simulink model "Drone_Simulation"  (R2020a)
settings: Solver=ode1  StartTime=0.0  StopTime=50  FixedStep=1e-3
values from neighbouring files (symbols this model uses):
  AeEMSC = 1    [Qball_X8_Model.m]
  alpha1TDDBSC = 1    [Qball_X8_Model.m]    (also in ReliabilityModel_Script.m = 0.7)
  bBNG = 1.2    [ReliabilityModel_Script.m]
  bEMSC = 1    [Qball_X8_Model.m]
  bEVCAP = 1    [Qball_X8_Model.m]    (also in ReliabilityModel_Script.m = 1.1)
  BNG_Motor1 = 0.8    [ReliabilityModel_Script.m]
  BNG_Motor2 = 1    [ReliabilityModel_Script.m]
  BNG_Motor3 = 1    [ReliabilityModel_Script.m]
  BNG_Motor4 = 1    [ReliabilityModel_Script.m]
  BNG_Motor5 = 1    [ReliabilityModel_Script.m]
  BNG_Motor6 = 1    [ReliabilityModel_Script.m]
  bp = 0.001    [ControlLawsScript.m]    (also in ControlLaws_Script.m)
  bq = 0.001    [ControlLawsScript.m]    (also in ControlLaws_Script.m)
  br = 0.001    [ControlLawsScript.m]    (also in ControlLaws_Script.m)
  bTDDBSC = 1    [Qball_X8_Model.m]    (also in ReliabilityModel_Script.m = 1.1)
  bWDG = 1    [Qball_X8_Model.m]    (also in ReliabilityModel_Script.m = 1.1)
  C_A = [     k_T           k_T          k_T                k_T          k_T         k_T ... (first row only)    [ControlLawsScript.m]    (also in ControlLaws_Script.m)
  C_mot = 1    [Qball_X8_Model.m]    (also in ReliabilityModel_Script.m = 17.46)
  C_th_esc = 1    [Qball_X8_Model.m]    (also in ReliabilityModel_Script.m = 1.67)
  CAPEV_Motor1 = 0.8    [ReliabilityModel_Script.m]
  CAPEV_Motor2 = 1    [ReliabilityModel_Script.m]
  CAPEV_Motor3 = 1    [ReliabilityModel_Script.m]
  CAPEV_Motor4 = 1    [ReliabilityModel_Script.m]
  CAPEV_Motor5 = 1    [ReliabilityModel_Script.m]
  CAPEV_Motor6 = 1    [ReliabilityModel_Script.m]
  cdx = cx*m    (= 17.4057414746)    [ControlLawsScript.m]    (also in ControlLaws_Script.m)
  cdy = cy*m    (= 17.4057414746)    [ControlLawsScript.m]    (also in ControlLaws_Script.m)
  cdz = cz*m    (= 17.4057414746)    [ControlLawsScript.m]    (also in ControlLaws_Script.m)
  EaEMSC = 1    [Qball_X8_Model.m]
  EaEVCAP = 1    [Qball_X8_Model.m]    (also in ReliabilityModel_Script.m = 0.94)
  EalphaTDDBSC = 1    [Qball_X8_Model.m]    (also in ReliabilityModel_Script.m = 0.7)
  EaTDDBSC = 1    [Qball_X8_Model.m]    (also in ReliabilityModel_Script.m = 0.7)
  EaWDG = 1    [Qball_X8_Model.m]    (also in ReliabilityModel_Script.m = 0.5)
  g = 9.80665    [ControlLawsScript.m]    (also in ControlLaws_Script.m; Qball_X8_Model.m = 9.87)
  JrefEMSC = 1    [Qball_X8_Model.m]
  Jz = 0.15887270137511    (= 0.158872701375)    [ControlLawsScript.m]    (also in ControlLaws_Script.m)
  k_b = 1    [Qball_X8_Model.m]    (also in ReliabilityModel_Script.m = -21.8546)
  Kp = (Jx/Tc)-bp    (= 4.11390529802)    [ControlLawsScript.m]    (also in ControlLaws_Script.m)
  Kp2 = Jx*((4/ts))*((-4/ts)+((bp+Kp)/Jx))/Kp    (= 6.72163348437)    [ControlLawsScript.m]    (also in ControlLaws_Script.m)
  Kq = (Jy/Tc)-bq    (= 4.12186008142)    [ControlLawsScript.m]    (also in ControlLaws_Script.m)
  Kq2 = Jy*((4/ts))*((-4/ts)+((bq+Kq)/Jy))/Kq    (= 6.72163033191)    [ControlLawsScript.m]    (also in ControlLaws_Script.m)
  Kr = (Jz/(tsy/25))-br    (= 7.94263506876)    [ControlLawsScript.m]    (also in ControlLaws_Script.m)
  Kr2 = Jz*((4/tsy))*((-4/tsy)+((br+Kr)/Jz))/Kr    (= 6.72084606682)    [ControlLawsScript.m]    (also in ControlLaws_Script.m)
  kv = 1/930    (= 0.0010752688172)    [StingerScript.m]
  Kx = abs(Kx)    [ControlLawsScript.m]    (also in ControlLaws_Script.m)
  Ky = abs(Ky)    [ControlLawsScript.m]    (also in ControlLaws_Script.m)
  Kz = (m/Tcz)-cz    (= 38.5143536865)    [ControlLawsScript.m]    (also in ControlLaws_Script.m)
  Kz2 = m*((4/tsz))*((-4/tsz)+((cz+Kz)/m))/Kz    (= 1.89810050529)    [ControlLawsScript.m]    (also in ControlLaws_Script.m)
  LnomEMSC = 1    [Qball_X8_Model.m]
  LnomEVCAP = 1    [Qball_X8_Model.m]    (also in ReliabilityModel_Script.m = 10800000)
  LnomTDDBSC = 1    [Qball_X8_Model.m]    (also in ReliabilityModel_Script.m = 9997200)
  LnomWDG = 1    [Qball_X8_Model.m]    (also in ReliabilityModel_Script.m = 72000000)
  m = 3.4811482949175    (= 3.48114829492)    [ControlLawsScript.m]    (also in ControlLaws_Script.m; Qball_X8_Model.m = 1.45)
  max_yaw_moment = k_y*hov_thrust/k_T    (= 0.323744079512)    [ControlLawsScript.m]    (also in ControlLaws_Script.m = 0.57666914163)
  NEMSC = 1    [Qball_X8_Model.m]
  nEVCAP = 1    [Qball_X8_Model.m]    (also in ReliabilityModel_Script.m)
  pconst = 2    [Qball_X8_Model.m]    (also in ReliabilityModel_Script.m)
  pitch_angle_limit = 32/R2D    (= 0.558505360638)    [ControlLawsScript.m]    (also in ControlLaws_Script.m)
  R2D = 180/pi    (= 57.2957795131)    [ControlLawsScript.m]    (also in ControlLaws_Script.m)
  R_th_esc = 1    [Qball_X8_Model.m]    (also in ReliabilityModel_Script.m = 5.14)
  R_th_mot = 1    [Qball_X8_Model.m]    (also in ReliabilityModel_Script.m = 8.59)
  Re = 0.008    [Qball_X8_Model.m]    (also in ReliabilityModel_Script.m)
  roll_angle_limit = 32/R2D    (= 0.558505360638)    [ControlLawsScript.m]    (also in ControlLaws_Script.m)
  RrefBNG = 0.9    [ReliabilityModel_Script.m]
  RrefEMSC = 1    [Qball_X8_Model.m]
  RrefEVCAP = 1    [Qball_X8_Model.m]    (also in ReliabilityModel_Script.m = 0.9)
  RrefTDDBSC = 1    [Qball_X8_Model.m]    (also in ReliabilityModel_Script.m = 0.37)
  RrefWDG = 1    [Qball_X8_Model.m]    (also in ReliabilityModel_Script.m = 0.98)
  SCTDDB_Motor1 = 0.8    [ReliabilityModel_Script.m]
  SCTDDB_Motor2 = 1    [ReliabilityModel_Script.m]
  SCTDDB_Motor3 = 1    [ReliabilityModel_Script.m]
  SCTDDB_Motor4 = 1    [ReliabilityModel_Script.m]
  SCTDDB_Motor5 = 1    [ReliabilityModel_Script.m]
  SCTDDB_Motor6 = 1    [ReliabilityModel_Script.m]
  T_amb = 1    [Qball_X8_Model.m]    (also in ReliabilityModel_Script.m = 20)
  T_amb_mot = 1    [Qball_X8_Model.m]    (also in ReliabilityModel_Script.m = 20)
  t_D_SCTDDB = 30    [ReliabilityModel_Script.m]
  TrefEMSC = 1    [Qball_X8_Model.m]
  TrefEVCAP = 1    [Qball_X8_Model.m]    (also in ReliabilityModel_Script.m = 105)
  TrefTDDBSC = 1    [Qball_X8_Model.m]    (also in ReliabilityModel_Script.m = 150)
  TrefWDG = 1    [Qball_X8_Model.m]    (also in ReliabilityModel_Script.m = 40)
  Ub = 12    [Qball_X8_Model.m]    (also in ReliabilityModel_Script.m)
  VmaxEVCAP = 1    [Qball_X8_Model.m]    (also in ReliabilityModel_Script.m = 35)
  VnomEVCAP = 1    [Qball_X8_Model.m]    (also in ReliabilityModel_Script.m = 35)
  WDG_Motor1 = 0.8    [ReliabilityModel_Script.m]
  WDG_Motor2 = 1    [ReliabilityModel_Script.m]
  WDG_Motor3 = 1    [ReliabilityModel_Script.m]
  WDG_Motor4 = 1    [ReliabilityModel_Script.m]
  WDG_Motor5 = 1    [ReliabilityModel_Script.m]
  WDG_Motor6 = 1    [ReliabilityModel_Script.m]
  z_x = cx    (= 5)    [ControlLawsScript.m]    (also in ControlLaws_Script.m)
  z_y = cy    (= 5)    [ControlLawsScript.m]    (also in ControlLaws_Script.m)
undefined symbols (not defined in the file or in its folder): FuselageContactForces, LeftAftArm, LeftAftSkid, LeftArm, LeftFrontArm, LeftFrontSkid, LeftSideContactForces, Lower, missionPlanX, missionPlanY, missionPlanYaw, missionPlanZ, Newton, Raphson, RightAftArm, RightAftSkid, RightArm, RightFrontArm, RightFrontSkid, RightSideContactForces, SkidsContactForces, timeConstant, Upper, X, Y, Z
libraries: sm_lib x90, nesl_utility x78, fl_lib x61, ee_lib x19, dspinverses x1, dspmtrx3 x1
(part 5 of 5)

== system Drone_Simulation/PLANT MODEL/PROPELLER AND ARMS/Arms ==
  Arm {1..6} (6 alike) : sm_lib/Body Elements/File Solid  ExtGeomFileName=STL files\Arm.stl  UnitType=Custom  ExtGeomFileUnits=mm  StepReaderType=HEX  ExportConvexHullGeometry=on  InertiaType=CalculateFromGeometry  Mass=1  MassUnits=kg  CenterOfMass=[0 0 0]  CenterOfMassUnits=m  MomentsOfInertia=[1 1 1]  MomentsOfInertiaUnits=kg*m^2  ProductsOfInertia=[0 0 0]  ProductsOfInertiaUnits=kg*m^2  BasedOnType=Density  Density=rho1  DensityUnits=kg/m^3  DoExposeReferenceFrame=on  SerializedFrames=<Frames/>  GraphicType=FromGeometry  MarkerShape=Sphere  MarkerSize=10  GraphicVisPropType=SimpleVisualProperties  GraphicDiffuseColor=rgb1  GraphicSpecularColor=[0.5 0.5 0.5 1.0]  GraphicAmbientColor=[0.15 0.15 0.15 1.0]  GraphicEmissiveColor=[0.0 0.0 0.0 1.0]  GraphicShininess=75  GraphicOpacity=op1
  Left Contact Arms : SimscapeBus  HierarchyStrings=LeftFrontArm;LeftArm;LeftAftArm
  Motor {1..6} (6 alike) : sm_lib/Body Elements/File Solid  ExtGeomFileName=STL files\Motor.stp  UnitType=FromFile  ExtGeomFileUnits=mm  StepReaderType=HEX  ExportConvexHullGeometry=off  InertiaType=CalculateFromGeometry  Mass=1  MassUnits=kg  CenterOfMass=[0 0 0]  CenterOfMassUnits=m  MomentsOfInertia=[1 1 1]  MomentsOfInertiaUnits=kg*m^2  ProductsOfInertia=[0 0 0]  ProductsOfInertiaUnits=kg*m^2  BasedOnType=Density  Density=rhoM  DensityUnits=kg/m^3  DoExposeReferenceFrame=on  SerializedFrames=<Frames/>  GraphicType=FromGeometry  MarkerShape=Sphere  MarkerSize=10  GraphicVisPropType=SimpleVisualProperties  GraphicDiffuseColor=[0.5 0.5 0.5]  GraphicSpecularColor=[0.5 0.5 0.5 1.0]  GraphicAmbientColor=[0.15 0.15 0.15 1.0]  GraphicEmissiveColor=[0.0 0.0 0.0 1.0]  GraphicShininess=75  GraphicOpacity=1.0
  Right Contact Arms : SimscapeBus  HierarchyStrings=RightFrontArm;RightArm;RightAftArm
  Rigid Transform{,6..10} (6 alike) : sm_lib/Frames and Transforms/Rigid Transform  TranslationMethod=Cartesian  TranslationStandardOffset=0  TranslationLengthUnit=m  TranslationStandardAxis=+Z  TranslationCartesianOffset=[0 0.3805 0.017]  TranslationROffset=0  TranslationROffsetUnits=m  TranslationZOffset=0  TranslationZOffsetUnits=m  TranslationThetaOffset=0  TranslationThetaOffsetUnits=deg  RotationMethod=StandardAxis  RotationAngleUnits=deg  RotationStandardAxis=-X  RotationAngle=180  RotationArbitraryAxis=[0 0 1]  FollAlignAxisA=+X  BaseAlignAxisA=+Y  FollAlignAxisB=+Y  BaseAlignAxisB=+Z  RotationSequenceAxes=FollowerAxes  RotationSequence=XYX  RotationSequenceAngles=[0 0 0]  RotationSequenceAnglesUnits=deg  RotationMatrix=[1 0 0; 0 1 0; 0 0 1]
  Rigid Transform1 : sm_lib/Frames and Transforms/Rigid Transform  TranslationMethod=Cartesian  TranslationStandardOffset=0  TranslationLengthUnit=m  TranslationStandardAxis=+Z  TranslationCartesianOffset=[0 0 0]  TranslationROffset=0  TranslationROffsetUnits=m  TranslationZOffset=0  TranslationZOffsetUnits=m  TranslationThetaOffset=0  TranslationThetaOffsetUnits=deg  RotationMethod=StandardAxis  RotationAngleUnits=deg  RotationStandardAxis=+Z  RotationAngle=0  RotationArbitraryAxis=[0 0 1]  FollAlignAxisA=+X  BaseAlignAxisA=+Y  FollAlignAxisB=+Y  BaseAlignAxisB=+Z  RotationSequenceAxes=FollowerAxes  RotationSequence=ZYX  RotationSequenceAngles=[0 0 0]  RotationSequenceAnglesUnits=deg  RotationMatrix=[1 0 0; 0 1 0; 0 0 1]
  Rigid Transform2 : sm_lib/Frames and Transforms/Rigid Transform  TranslationMethod=Cartesian  TranslationStandardOffset=0  TranslationLengthUnit=m  TranslationStandardAxis=+Z  TranslationCartesianOffset=[0 0 0]  TranslationROffset=0  TranslationROffsetUnits=m  TranslationZOffset=0  TranslationZOffsetUnits=m  TranslationThetaOffset=0  TranslationThetaOffsetUnits=deg  RotationMethod=StandardAxis  RotationAngleUnits=deg  RotationStandardAxis=+Z  RotationAngle=60  RotationArbitraryAxis=[0 0 1]  FollAlignAxisA=+X  BaseAlignAxisA=+Y  FollAlignAxisB=+Y  BaseAlignAxisB=+Z  RotationSequenceAxes=FollowerAxes  RotationSequence=ZYX  RotationSequenceAngles=[0 0 0]  RotationSequenceAnglesUnits=deg  RotationMatrix=[1 0 0; 0 1 0; 0 0 1]
  Rigid Transform3 : sm_lib/Frames and Transforms/Rigid Transform  TranslationMethod=Cartesian  TranslationStandardOffset=0  TranslationLengthUnit=m  TranslationStandardAxis=+Z  TranslationCartesianOffset=[0 0 0]  TranslationROffset=0  TranslationROffsetUnits=m  TranslationZOffset=0  TranslationZOffsetUnits=m  TranslationThetaOffset=0  TranslationThetaOffsetUnits=deg  RotationMethod=StandardAxis  RotationAngleUnits=deg  RotationStandardAxis=+Z  RotationAngle=120  RotationArbitraryAxis=[0 0 1]  FollAlignAxisA=+X  BaseAlignAxisA=+Y  FollAlignAxisB=+Y  BaseAlignAxisB=+Z  RotationSequenceAxes=FollowerAxes  RotationSequence=ZYX  RotationSequenceAngles=[0 0 0]  RotationSequenceAnglesUnits=deg  RotationMatrix=[1 0 0; 0 1 0; 0 0 1]
  Rigid Transform4 : sm_lib/Frames and Transforms/Rigid Transform  TranslationMethod=Cartesian  TranslationStandardOffset=0  TranslationLengthUnit=m  TranslationStandardAxis=+Z  TranslationCartesianOffset=[0 0 0]  TranslationROffset=0  TranslationROffsetUnits=m  TranslationZOffset=0  TranslationZOffsetUnits=m  TranslationThetaOffset=0  TranslationThetaOffsetUnits=deg  RotationMethod=StandardAxis  RotationAngleUnits=deg  RotationStandardAxis=+Z  RotationAngle=180  RotationArbitraryAxis=[0 0 1]  FollAlignAxisA=+X  BaseAlignAxisA=+Y  FollAlignAxisB=+Y  BaseAlignAxisB=+Z  RotationSequenceAxes=FollowerAxes  RotationSequence=ZYX  RotationSequenceAngles=[0 0 0]  RotationSequenceAnglesUnits=deg  RotationMatrix=[1 0 0; 0 1 0; 0 0 1]
  Rigid Transform5 : sm_lib/Frames and Transforms/Rigid Transform  TranslationMethod=Cartesian  TranslationStandardOffset=0  TranslationLengthUnit=m  TranslationStandardAxis=+Z  TranslationCartesianOffset=[0 0 0]  TranslationROffset=0  TranslationROffsetUnits=m  TranslationZOffset=0  TranslationZOffsetUnits=m  TranslationThetaOffset=0  TranslationThetaOffsetUnits=deg  RotationMethod=StandardAxis  RotationAngleUnits=deg  RotationStandardAxis=+Z  RotationAngle=240  RotationArbitraryAxis=[0 0 1]  FollAlignAxisA=+X  BaseAlignAxisA=+Y  FollAlignAxisB=+Y  BaseAlignAxisB=+Z  RotationSequenceAxes=FollowerAxes  RotationSequence=ZYX  RotationSequenceAngles=[0 0 0]  RotationSequenceAnglesUnits=deg  RotationMatrix=[1 0 0; 0 1 0; 0 0 1]
  Rigid Transform62 : sm_lib/Frames and Transforms/Rigid Transform  TranslationMethod=Cartesian  TranslationStandardOffset=0  TranslationLengthUnit=m  TranslationStandardAxis=+Z  TranslationCartesianOffset=[0 0 0]  TranslationROffset=0  TranslationROffsetUnits=m  TranslationZOffset=0  TranslationZOffsetUnits=m  TranslationThetaOffset=0  TranslationThetaOffsetUnits=deg  RotationMethod=StandardAxis  RotationAngleUnits=deg  RotationStandardAxis=+Z  RotationAngle=300  RotationArbitraryAxis=[0 0 1]  FollAlignAxisA=+X  BaseAlignAxisA=+Y  FollAlignAxisB=+Y  BaseAlignAxisB=+Z  RotationSequenceAxes=FollowerAxes  RotationSequence=ZYX  RotationSequenceAngles=[0 0 0]  RotationSequenceAnglesUnits=deg  RotationMatrix=[1 0 0; 0 1 0; 0 0 1]
  Left-Front : PMIOPort  Side=Left
  Right-Front : PMIOPort  Port=2  Side=Left
  Left : PMIOPort  Port=3  Side=Left
  Right : PMIOPort  Port=4  Side=Left
  Left-Aft : PMIOPort  Port=5  Side=Left
  Right-Aft : PMIOPort  Port=6  Side=Left
  Fuselage : PMIOPort  Port=7  Side=Left
  Left Contact : PMIOPort  Port=8  Side=Right
  Right Contact : PMIOPort  Port=9  Side=Right
  connections:
  Right-Front/RConn1 -- Arm 1/RConn1 -- Rigid Transform7/LConn1 -- Rigid Transform5/RConn1
  Left-Front/RConn1 -- Arm 6/RConn1 -- Rigid Transform10/LConn1 -- Rigid Transform62/RConn1
  Right-Aft/RConn1 -- Arm 3/RConn1 -- Rigid Transform/LConn1 -- Rigid Transform3/RConn1
  Left-Aft/RConn1 -- Arm 4/RConn1 -- Rigid Transform8/LConn1 -- Rigid Transform2/RConn1
  Left/RConn1 -- Rigid Transform1/RConn1 -- Arm 5/RConn1 -- Rigid Transform9/LConn1
  Rigid Transform1/LConn1 -- Rigid Transform62/LConn1 -- Rigid Transform5/LConn1 -- Rigid Transform4/LConn1 -- Rigid Transform3/LConn1 -- Rigid Transform2/LConn1 -- Fuselage/RConn1
  Right/RConn1 -- Arm 2/RConn1 -- Rigid Transform6/LConn1 -- Rigid Transform4/RConn1
  Right Contact/RConn1 -- Right Contact Arms/RConn1
  Arm 5/LConn1 -- Left Contact Arms/LConn2
  Arm 2/LConn1 -- Right Contact Arms/LConn2
  Arm 3/LConn1 -- Right Contact Arms/LConn3
  Arm 1/LConn1 -- Right Contact Arms/LConn1
  Arm 6/LConn1 -- Left Contact Arms/LConn1
  Arm 4/LConn1 -- Left Contact Arms/LConn3
  Left Contact/RConn1 -- Left Contact Arms/RConn1
  Motor 3/RConn1 -- Rigid Transform/RConn1
  Motor 2/RConn1 -- Rigid Transform6/RConn1
  Motor 1/RConn1 -- Rigid Transform7/RConn1
  Motor 4/RConn1 -- Rigid Transform8/RConn1
  Motor 5/RConn1 -- Rigid Transform9/RConn1
  Motor 6/RConn1 -- Rigid Transform10/RConn1

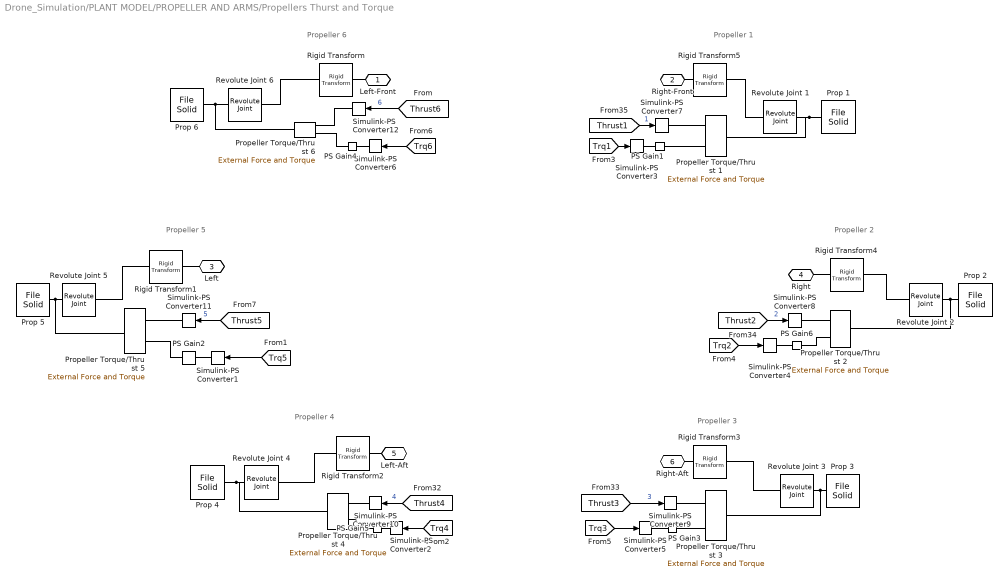
== system Drone_Simulation/PLANT MODEL/PROPELLER AND ARMS/Propellers Thurst and Torque ==
  note: Propeller 1
  note: Propeller 2
  note: Propeller 3
  note: Propeller 4
  note: Propeller 5
  note: Propeller 6
  PS Gain1 : fl_lib/Physical Signals/Functions/PS Gain  gain=-1
  PS Gain2 : fl_lib/Physical Signals/Functions/PS Gain  gain=-1
  PS Gain3 : fl_lib/Physical Signals/Functions/PS Gain  gain=-1
  PS Gain4 : fl_lib/Physical Signals/Functions/PS Gain  gain=1
  PS Gain5 : fl_lib/Physical Signals/Functions/PS Gain  gain=1
  PS Gain6 : fl_lib/Physical Signals/Functions/PS Gain  gain=1
  Prop {1..3,6} (4 alike) : sm_lib/Body Elements/File Solid  ExtGeomFileName=STL files\Propeller.stl  UnitType=Custom  ExtGeomFileUnits=m  StepReaderType=HEX  ExportConvexHullGeometry=off  InertiaType=CalculateFromGeometry  Mass=1  MassUnits=kg  CenterOfMass=[0 0 0]  CenterOfMassUnits=m  MomentsOfInertia=[1 1 1]  MomentsOfInertiaUnits=kg*m^2  ProductsOfInertia=[0 0 0]  ProductsOfInertiaUnits=kg*m^2  BasedOnType=Density  Density=rhoP  DensityUnits=kg/m^3  DoExposeReferenceFrame=on  SerializedFrames=<Frames/>  GraphicType=FromGeometry  MarkerShape=Sphere  MarkerSize=10  GraphicVisPropType=SimpleVisualProperties  GraphicDiffuseColor=rgbP  GraphicSpecularColor=[0.5 0.5 0.5 1.0]  GraphicAmbientColor=[0.15 0.15 0.15 1.0]  GraphicEmissiveColor=[0.0 0.0 0.0 1.0]  GraphicShininess=75  GraphicOpacity=opP
  Prop 4 : sm_lib/Body Elements/File Solid  ExtGeomFileName=STL files\Propeller.stl  UnitType=Custom  ExtGeomFileUnits=m  StepReaderType=HEX  ExportConvexHullGeometry=off  InertiaType=CalculateFromGeometry  Mass=1  MassUnits=kg  CenterOfMass=[0 0 0.1]  CenterOfMassUnits=m  MomentsOfInertia=[1 1 1]  MomentsOfInertiaUnits=kg*m^2  ProductsOfInertia=[0 0 0]  ProductsOfInertiaUnits=kg*m^2  BasedOnType=Density  Density=rhoP  DensityUnits=kg/m^3  DoExposeReferenceFrame=on  SerializedFrames=<Frames/>  GraphicType=FromGeometry  MarkerShape=Sphere  MarkerSize=10  GraphicVisPropType=SimpleVisualProperties  GraphicDiffuseColor=rgbP  GraphicSpecularColor=[0.5 0.5 0.5 1.0]  GraphicAmbientColor=[0.15 0.15 0.15 1.0]  GraphicEmissiveColor=[0.0 0.0 0.0 1.0]  GraphicShininess=75  GraphicOpacity=opP
  Prop 5 : sm_lib/Body Elements/File Solid  ExtGeomFileName=STL files\Propeller.stl  UnitType=Custom  ExtGeomFileUnits=m  StepReaderType=HEX  ExportConvexHullGeometry=off  InertiaType=CalculateFromGeometry  Mass=1  MassUnits=kg  CenterOfMass=[0 0 0.1]  CenterOfMassUnits=m  MomentsOfInertia=[1 1 1]  MomentsOfInertiaUnits=kg*m^2  ProductsOfInertia=[0 0 0]  ProductsOfInertiaUnits=kg*m^2  BasedOnType=Density  Density=rhoP  DensityUnits=kg/m^3  DoExposeReferenceFrame=on  SerializedFrames=<Frames/>  GraphicType=FromGeometry  MarkerShape=Sphere  MarkerSize=10  GraphicVisPropType=SimpleVisualProperties  GraphicDiffuseColor=rgbP  GraphicSpecularColor=[0.5 0.5 0.5 1.0]  GraphicAmbientColor=[0.15 0.15 0.15 1.0]  GraphicEmissiveColor=[0.0 0.0 0.0 1.0]  GraphicShininess=75  GraphicOpacity=opP
  Propeller Torque/Thrust {1..6} (6 alike) : sm_lib/Forces and Torques/External Force and Torque  ForceResolutionFrame=AttachedFrame  EnableForceX=off  EnableForceY=off  EnableForceZ=on  EnableForce=off  TorqueResolutionFrame=AttachedFrame  EnableTorqueX=off  EnableTorqueY=off  EnableTorqueZ=on  EnableTorque=off
  Revolute Joint {1..6} (6 alike) : sm_lib/Joints/Revolute Joint  JointMode=Normal  SenseConstraintForce=off  SenseConstraintForceX=off  SenseConstraintForceY=off  SenseConstraintForceZ=off  SenseConstraintTorque=off  SenseConstraintTorqueX=off  SenseConstraintTorqueY=off  SenseConstraintTorqueZ=off  SenseTotalForce=off  SenseTotalForceX=off  SenseTotalForceY=off  SenseTotalForceZ=off  SenseTotalTorque=off  SenseTotalTorqueX=off  SenseTotalTorqueY=off  SenseTotalTorqueZ=off  CompositeWrenchDir=FollowerOnBase  CompositeWrenchFrame=BaseFrame  EquilibriumPosition=0  EquilibriumPositionUnits=deg  SpringStiffness=0  SpringStiffnessUnits=N*m/deg  DampingCoefficient=br/Jz  DampingCoefficientUnits=N*m/(rad/s)  TorqueActuationMode=NoTorque  MotionActuationMode=ComputedMotion  SensePosition=off  SenseVelocity=off  SenseAcceleration=off  SenseTorqueForce=off  SenseLowerLimitTorqueForce=off  SenseUpperLimitTorqueForce=off  LowerLimitSpecify=off  LowerLimitBound=-90  LowerLimitBoundUnits=deg  LowerLimitStiffness=1e4  LowerLimitStiffnessUnits=N*m/deg  LowerLimitDamping=10  LowerLimitDampingUnits=N*m/(deg/s)  LowerLimitTransitionRegionWidth=0.1  LowerLimitTransitionRegionWidthUnits=deg  UpperLimitSpecify=off  UpperLimitBound=90  UpperLimitBoundUnits=deg  UpperLimitStiffness=1e4  UpperLimitStiffnessUnits=N*m/deg  UpperLimitDamping=10  UpperLimitDampingUnits=N*m/(deg/s)  UpperLimitTransitionRegionWidth=0.1  UpperLimitTransitionRegionWidthUnits=deg  PositionTargetSpecify=off  PositionTargetPriority=High  PositionTargetValue=0  PositionTargetValueUnits=deg  VelocityTargetSpecify=off  VelocityTargetPriority=High  VelocityTargetValue=0  VelocityTargetValueUnits=deg/s
  Rigid Transform{,1..5} (6 alike) : sm_lib/Frames and Transforms/Rigid Transform  TranslationMethod=Cartesian  TranslationStandardOffset=0  TranslationLengthUnit=m  TranslationStandardAxis=+Z  TranslationCartesianOffset=[0 -0.3805 -0.0375]  TranslationROffset=0  TranslationROffsetUnits=m  TranslationZOffset=0  TranslationZOffsetUnits=m  TranslationThetaOffset=0  TranslationThetaOffsetUnits=deg  RotationMethod=None  RotationAngleUnits=deg  RotationStandardAxis=+Z  RotationAngle=0.0  RotationArbitraryAxis=[0 0 1]  FollAlignAxisA=+X  BaseAlignAxisA=+Y  FollAlignAxisB=+Y  BaseAlignAxisB=+Z  RotationSequenceAxes=FollowerAxes  RotationSequence=XYX  RotationSequenceAngles=[0 0 0]  RotationSequenceAnglesUnits=deg  RotationMatrix=[1 0 0; 0 1 0; 0 0 1]
  Simulink-PS Converter{1..3,6} (4 alike) : nesl_utility/Simulink-PS Converter  PhysicalDomain=network_engine_domain  SubClassName=ps_input  LeftPortType=input  RightPortType=output  PseudoPeriodic=off  Frequencies=[]  NoiseDistribution=none  NoiseParameters=[]  Unit=N*m  AffineConversion=off  FilteringAndDerivatives=provide  SimscapeFilterOrder=2  InputFilterTimeConstant=0.001  UdotUserProvided=0
  Simulink-PS Converter{7..12} (6 alike) : nesl_utility/Simulink-PS Converter  PhysicalDomain=network_engine_domain  SubClassName=ps_input  LeftPortType=input  RightPortType=output  PseudoPeriodic=off  Frequencies=[]  NoiseDistribution=none  NoiseParameters=[]  Unit=1  AffineConversion=on  FilteringAndDerivatives=provide  SimscapeFilterOrder=2  InputFilterTimeConstant=0.001  UdotUserProvided=0
  Simulink-PS Converter4 : nesl_utility/Simulink-PS Converter  PhysicalDomain=network_engine_domain  SubClassName=ps_input  LeftPortType=input  RightPortType=output  PseudoPeriodic=off  Frequencies=[]  NoiseDistribution=none  NoiseParameters=[]  Unit=N*m  AffineConversion=on  FilteringAndDerivatives=provide  SimscapeFilterOrder=2  InputFilterTimeConstant=0.001  UdotUserProvided=0
  Simulink-PS Converter5 : nesl_utility/Simulink-PS Converter  PhysicalDomain=network_engine_domain  SubClassName=ps_input  LeftPortType=input  RightPortType=output  PseudoPeriodic=off  Frequencies=[]  NoiseDistribution=none  NoiseParameters=[]  Unit=N*m  AffineConversion=on  FilteringAndDerivatives=provide  SimscapeFilterOrder=2  InputFilterTimeConstant=0.001  UdotUserProvided=0
  Left-Front : PMIOPort  Side=Right
  Right-Front : PMIOPort  Port=2  Side=Right
  Left : PMIOPort  Port=3  Side=Right
  Right : PMIOPort  Port=4  Side=Right
  Left-Aft : PMIOPort  Port=5  Side=Right
  Right-Aft : PMIOPort  Port=6  Side=Right
  wires:
  [Trq4] -> Simulink-PS Converter2/1
  [Trq5] -> Simulink-PS Converter1/1
  [Trq6] -> Simulink-PS Converter6/1
  [Trq1] -> Simulink-PS Converter3/1
  [Trq3] -> Simulink-PS Converter5/1
  [Trq2] -> Simulink-PS Converter4/1
  [Thrust1] -> Simulink-PS Converter7/1  "1"
  [Thrust2] -> Simulink-PS Converter8/1  "2"
  [Thrust3] -> Simulink-PS Converter9/1  "3"
  [Thrust4] -> Simulink-PS Converter10/1  "4"
  [Thrust5] -> Simulink-PS Converter11/1  "5"
  [Thrust6] -> Simulink-PS Converter12/1  "6"
  connections:
  Revolute Joint 2/RConn1 -- Propeller Torque/Thrust 2/RConn1 -- Prop 2/RConn1
  Rigid Transform5/RConn1 -- Right-Front/RConn1
  Rigid Transform5/LConn1 -- Revolute Joint 1/LConn1
  Revolute Joint 3/RConn1 -- Propeller Torque/Thrust 3/RConn1 -- Prop 3/RConn1
  Rigid Transform4/RConn1 -- Right/RConn1
  Rigid Transform4/LConn1 -- Revolute Joint 2/LConn1
  Rigid Transform3/RConn1 -- Right-Aft/RConn1
  Rigid Transform/RConn1 -- Left-Front/RConn1
  Simulink-PS Converter3/RConn1 -- PS Gain1/LConn1
  Simulink-PS Converter1/RConn1 -- PS Gain2/LConn1
  Simulink-PS Converter5/RConn1 -- PS Gain3/LConn1
  Simulink-PS Converter6/RConn1 -- PS Gain4/LConn1
  Simulink-PS Converter2/RConn1 -- PS Gain5/LConn1
  Simulink-PS Converter4/RConn1 -- PS Gain6/LConn1
  Rigid Transform2/RConn1 -- Left-Aft/RConn1
  Rigid Transform1/RConn1 -- Left/RConn1
  Prop 6/RConn1 -- Propeller Torque/Thrust 6/RConn1 -- Revolute Joint 6/RConn1
  Revolute Joint 1/RConn1 -- Propeller Torque/Thrust 1/RConn1 -- Prop 1/RConn1
  Revolute Joint 4/RConn1 -- Propeller Torque/Thrust 4/RConn1 -- Prop 4/RConn1
  Revolute Joint 5/RConn1 -- Propeller Torque/Thrust 5/RConn1 -- Prop 5/RConn1
  Rigid Transform2/LConn1 -- Revolute Joint 4/LConn1
  Rigid Transform1/LConn1 -- Revolute Joint 5/LConn1
  Rigid Transform3/LConn1 -- Revolute Joint 3/LConn1
  Rigid Transform/LConn1 -- Revolute Joint 6/LConn1
  Simulink-PS Converter8/RConn1 -- Propeller Torque/Thrust 2/LConn1
  PS Gain6/RConn1 -- Propeller Torque/Thrust 2/LConn2
  Propeller Torque/Thrust 3/LConn2 -- PS Gain3/RConn1
  Simulink-PS Converter9/RConn1 -- Propeller Torque/Thrust 3/LConn1
  Simulink-PS Converter10/RConn1 -- Propeller Torque/Thrust 4/LConn1
  PS Gain5/RConn1 -- Propeller Torque/Thrust 4/LConn2
  PS Gain2/RConn1 -- Propeller Torque/Thrust 5/LConn2
  Simulink-PS Converter11/RConn1 -- Propeller Torque/Thrust 5/LConn1
  Simulink-PS Converter12/RConn1 -- Propeller Torque/Thrust 6/LConn1
  PS Gain4/RConn1 -- Propeller Torque/Thrust 6/LConn2
  Simulink-PS Converter7/RConn1 -- Propeller Torque/Thrust 1/LConn1
  PS Gain1/RConn1 -- Propeller Torque/Thrust 1/LConn2

== system Drone_Simulation/PLANT MODEL/SENSORS/Quaternion to Rotation Angles, XYZ order ==
  note: Protect asincos input
  note: Angle Calculation
  q : Inport  Unit=1
  Demux : Demux
  Demux1 : Demux
  If : If  IfExpression=u1 > 1  ElseIfExpressions=u1 < -1
  If Action Subsystem : Subsystem  TreatAsAtomicUnit=on
  If Action Subsystem1 : Subsystem  TreatAsAtomicUnit=on
  If Action Subsystem2 : Subsystem  TreatAsAtomicUnit=on
  Merge : Merge  Inputs=3
  Mux : Mux
  Product{,1..3} (4 alike) : Product  Inputs=*/
  Product{4..7} (4 alike) : Product
  Sum : Sum  Inputs=4
  Trigonometric Function1 : Trigonometry  Operator=atan2
  Trigonometric Function3 : Trigonometry  Operator=atan2
  Vector Concatenate : Concatenate  NumInputs=3
  fcn1 : Fcn  Expr=2*(u[2]*u[3] + u[1]*u[4])
  fcn2 : Fcn  Expr=u[1]*u[1] + u[2]*u[2] - u[3]*u[3] - u[4]*u[4]
  fcn3 : Fcn  Expr=-2*(u[2]*u[4] - u[1]*u[3])
  fcn4 : Fcn  Expr=2*(u[3]*u[4] + u[1]*u[2])
  fcn5 : Fcn  Expr=u[1]*u[1] - u[2]*u[2] - u[3]*u[3] + u[4]*u[4]
  sqrt : Sqrt  AlgorithmType=Newton-Raphson  SaturateOnIntegerOverflow=on
  trigFcn : Trigonometry  Operator=asin
  R1,R2,R3 : Outport  Unit=rad  VectorParamsAs1DForOutWhenUnconnected=off
  wires:
  Mux/1 -> fcn5/1, fcn4/1, fcn2/1, fcn1/1, fcn3/1
  Vector Concatenate/1 -> R1,R2,R3/1
  trigFcn/1 -> Vector Concatenate/2  "r2"
  Trigonometric Function1/1 -> Vector Concatenate/1  "r1"
  fcn2/1 -> Trigonometric Function1/2
  fcn4/1 -> Trigonometric Function3/1
  Trigonometric Function3/1 -> Vector Concatenate/3  "r3"
  fcn1/1 -> Trigonometric Function1/1
  fcn5/1 -> Trigonometric Function3/2
  Merge/1 -> trigFcn/1
  If/1 -> If Action Subsystem/Action
  fcn3/1 -> If/1, If Action Subsystem2/1(In)
  If/2 -> If Action Subsystem1/Action
  If/3 -> If Action Subsystem2/Action
  If Action Subsystem/1(OutputPos1) -> Merge/1
  If Action Subsystem1/1(OutputNeg1) -> Merge/2
  If Action Subsystem2/1(OutOrig) -> Merge/3
  Demux/2 -> Product1/1
  sqrt/1 -> Product3/2, Product2/2, Product/2, Product1/2
  Demux/1 -> Product/1
  Demux/4 -> Product3/1
  Product2/1 -> Mux/3
  Product/1 -> Mux/1
  Product1/1 -> Mux/2
  Demux/3 -> Product2/1
  Product3/1 -> Mux/4
  Sum/1 -> sqrt/1
  q/1 -> Demux/1, Demux1/1
  Demux1/2 -> Product5/1, Product5/2
  Product7/1 -> Sum/4
  Demux1/3 -> Product6/1, Product6/2
  Product5/1 -> Sum/2
  Demux1/4 -> Product7/1, Product7/2
  Product4/1 -> Sum/1
  Demux1/1 -> Product4/1, Product4/2
  Product6/1 -> Sum/3

== system Drone_Simulation/PLANT MODEL/ELECTRIC SYSTEM/Motor 1/RPM to Resistive Torque and Thrust1 ==
  Angular Speed : Inport
  Gain : Gain  Gain=-1
  Math Function : Math  Operator=square  SaturateOnIntegerOverflow=on
  Math Function1 : Math  Operator=square  SaturateOnIntegerOverflow=on
  Math Function2 : Math  Operator=square  SaturateOnIntegerOverflow=on
  Square Root : Sqrt  SaturateOnIntegerOverflow=on
  Sum : Sum  Inputs=+++
  Thrust & Torque Based on Propeller Rotational and Translational Velocity : MATLAB Function  TreatAsAtomicUnit=on
  Thrust : Outport
  Resistive Torque : Outport  Port=2
  wires:
  Gain/1 -> Resistive Torque/1
  Square Root/1 -> Thrust & Torque Based on Propeller Rotational and Translational Velocity/1(Velocity)
  Thrust & Torque Based on Propeller Rotational and Translational Velocity/2(Torque) -> Gain/1
  Angular Speed/1 -> Thrust & Torque Based on Propeller Rotational and Translational Velocity/2(RPM)  "Speed"
  Thrust & Torque Based on Propeller Rotational and Translational Velocity/1(Thrust) -> Thrust/1
  [DX] -> Math Function/1
  [DY] -> Math Function1/1
  [DZ] -> Math Function2/1
  Math Function/1 -> Sum/1
  Math Function1/1 -> Sum/2
  Math Function2/1 -> Sum/3
  Sum/1 -> Square Root/1

== system Drone_Simulation/PLANT MODEL/ELECTRIC SYSTEM/Motor 1/Signals ==
  Mux : Mux  Inputs=2
      settings: DisplayOption=signals
  Spd : Outport  VectorParamsAs1DForOutWhenUnconnected=off
  ia : Outport  Port=2  VectorParamsAs1DForOutWhenUnconnected=off
  Trq : Outport  Port=3  VectorParamsAs1DForOutWhenUnconnected=off
  V : Outport  Port=4  VectorParamsAs1DForOutWhenUnconnected=off
  wires:
  [Trq1] -> Trq/1  "Motor torque [N*m]"
  [AngularSpeed1] -> Mux/2  "actual speed"
  Mux/1 -> Spd/1  "Requested and measured velocity [rpm]"
  [ReqSpeedMotor1] -> Mux/1  "req speed"
  [I_ESC_OUT1] -> ia/1  "Armature current [A]"
  [V_ESC_OUT1] -> V/1  "Motor Voltage (V)"

== system Drone_Simulation/PLANT MODEL/ELECTRIC SYSTEM/Motor 2/RPM to Resistive Torque and Thrust ==
  Angular Speed : Inport
  Gain : Gain  Gain=-1
  Math Function : Math  Operator=square  SaturateOnIntegerOverflow=on
  Math Function1 : Math  Operator=square  SaturateOnIntegerOverflow=on
  Math Function2 : Math  Operator=square  SaturateOnIntegerOverflow=on
  Square Root : Sqrt  SaturateOnIntegerOverflow=on
  Sum : Sum  Inputs=+++
  Thrust & Torque Based on Propeller Rotational and Translational Velocity : MATLAB Function  TreatAsAtomicUnit=on
  Thrust : Outport
  Resistive Torque : Outport  Port=2
  wires:
  Gain/1 -> Resistive Torque/1
  Thrust & Torque Based on Propeller Rotational and Translational Velocity/2(Torque) -> Gain/1
  Angular Speed/1 -> Thrust & Torque Based on Propeller Rotational and Translational Velocity/2(RPM)  "Speed"
  Thrust & Torque Based on Propeller Rotational and Translational Velocity/1(Thrust) -> Thrust/1
  [DX] -> Math Function/1
  Math Function/1 -> Sum/1
  Math Function2/1 -> Sum/3
  Sum/1 -> Square Root/1
  Math Function1/1 -> Sum/2
  [DZ] -> Math Function2/1
  [DY] -> Math Function1/1
  Square Root/1 -> Thrust & Torque Based on Propeller Rotational and Translational Velocity/1(Velocity)

== system Drone_Simulation/PLANT MODEL/ELECTRIC SYSTEM/Motor 2/Signals ==
  Mux : Mux  Inputs=2
      settings: DisplayOption=signals
  Spd : Outport  VectorParamsAs1DForOutWhenUnconnected=off
  ia : Outport  Port=2  VectorParamsAs1DForOutWhenUnconnected=off
  Trq : Outport  Port=3  VectorParamsAs1DForOutWhenUnconnected=off
  V : Outport  Port=4  VectorParamsAs1DForOutWhenUnconnected=off
  wires:
  [Trq2] -> Trq/1  "Motor torque [N*m]"
  [AngularSpeed2] -> Mux/2  "actual speed"
  Mux/1 -> Spd/1  "Requested and measured velocity [rpm]"
  [ReqSpeedMotor2] -> Mux/1  "req speed"
  [I_ESC_OUT2] -> ia/1  "Armature current [A]"
  [V_ESC_OUT2] -> V/1  "Motor Voltage (V)"

== system Drone_Simulation/PLANT MODEL/ELECTRIC SYSTEM/Motor 3/RPM to Resistive Torque and Thrust ==
  Angular Speed : Inport
  Gain : Gain  Gain=-1
  Math Function : Math  Operator=square  SaturateOnIntegerOverflow=on
  Math Function1 : Math  Operator=square  SaturateOnIntegerOverflow=on
  Math Function2 : Math  Operator=square  SaturateOnIntegerOverflow=on
  Square Root : Sqrt  SaturateOnIntegerOverflow=on
  Sum : Sum  Inputs=+++
  Thrust & Torque Based on Propeller Rotational and Translational Velocity : MATLAB Function  TreatAsAtomicUnit=on
  Thrust : Outport
  Resistive Torque : Outport  Port=2
  wires:
  Gain/1 -> Resistive Torque/1
  Thrust & Torque Based on Propeller Rotational and Translational Velocity/2(Torque) -> Gain/1
  Angular Speed/1 -> Thrust & Torque Based on Propeller Rotational and Translational Velocity/2(RPM)  "Speed"
  Thrust & Torque Based on Propeller Rotational and Translational Velocity/1(Thrust) -> Thrust/1
  [DX] -> Math Function/1
  Math Function/1 -> Sum/1
  Math Function2/1 -> Sum/3
  Sum/1 -> Square Root/1
  Square Root/1 -> Thrust & Torque Based on Propeller Rotational and Translational Velocity/1(Velocity)
  Math Function1/1 -> Sum/2
  [DZ] -> Math Function2/1
  [DY] -> Math Function1/1

== system Drone_Simulation/PLANT MODEL/ELECTRIC SYSTEM/Motor 3/Signals ==
  Mux : Mux  Inputs=2
      settings: DisplayOption=signals
  Spd : Outport  VectorParamsAs1DForOutWhenUnconnected=off
  ia : Outport  Port=2  VectorParamsAs1DForOutWhenUnconnected=off
  Trq : Outport  Port=3  VectorParamsAs1DForOutWhenUnconnected=off
  V : Outport  Port=4  VectorParamsAs1DForOutWhenUnconnected=off
  wires:
  [Trq3] -> Trq/1  "Motor torque [N*m]"
  [AngularSpeed3] -> Mux/2  "actual speed"
  Mux/1 -> Spd/1  "Requested and measured velocity [rpm]"
  [ReqSpeedMotor3] -> Mux/1  "req speed"
  [I_ESC_OUT3] -> ia/1  "Armature current [A]"
  [V_ESC_OUT3] -> V/1  "Motor Voltage (V)"

== system Drone_Simulation/PLANT MODEL/ELECTRIC SYSTEM/Motor 4/RPM to Resistive Torque and Thrust ==
  Angular Speed : Inport
  Gain : Gain  Gain=-1
  Math Function : Math  Operator=square  SaturateOnIntegerOverflow=on
  Math Function1 : Math  Operator=square  SaturateOnIntegerOverflow=on
  Math Function2 : Math  Operator=square  SaturateOnIntegerOverflow=on
  Square Root : Sqrt  SaturateOnIntegerOverflow=on
  Sum : Sum  Inputs=+++
  Thrust & Torque Based on Propeller Rotational and Translational Velocity : MATLAB Function  TreatAsAtomicUnit=on
  Thrust : Outport
  Resistive Torque : Outport  Port=2
  wires:
  Gain/1 -> Resistive Torque/1
  Thrust & Torque Based on Propeller Rotational and Translational Velocity/2(Torque) -> Gain/1
  Angular Speed/1 -> Thrust & Torque Based on Propeller Rotational and Translational Velocity/2(RPM)  "Speed"
  Thrust & Torque Based on Propeller Rotational and Translational Velocity/1(Thrust) -> Thrust/1
  [DX] -> Math Function/1
  Math Function/1 -> Sum/1
  Math Function2/1 -> Sum/3
  Sum/1 -> Square Root/1
  Square Root/1 -> Thrust & Torque Based on Propeller Rotational and Translational Velocity/1(Velocity)
  Math Function1/1 -> Sum/2
  [DZ] -> Math Function2/1
  [DY] -> Math Function1/1

== system Drone_Simulation/PLANT MODEL/ELECTRIC SYSTEM/Motor 4/Signals ==
  Mux : Mux  Inputs=2
      settings: DisplayOption=signals
  Spd : Outport  VectorParamsAs1DForOutWhenUnconnected=off
  ia : Outport  Port=2  VectorParamsAs1DForOutWhenUnconnected=off
  Trq : Outport  Port=3  VectorParamsAs1DForOutWhenUnconnected=off
  V : Outport  Port=4  VectorParamsAs1DForOutWhenUnconnected=off
  wires:
  [Trq4] -> Trq/1  "Motor torque [N*m]"
  [AngularSpeed4] -> Mux/2  "actual speed"
  Mux/1 -> Spd/1  "Requested and measured velocity [rpm]"
  [ReqSpeedMotor4] -> Mux/1  "req speed"
  [I_ESC_OUT4] -> ia/1  "Armature current [A]"
  [V_ESC_OUT4] -> V/1  "Motor Voltage (V)"

== system Drone_Simulation/PLANT MODEL/ELECTRIC SYSTEM/Motor 5/RPM to Resistive Torque and Thrust ==
  Angular Speed : Inport
  Gain : Gain  Gain=-1
  Math Function : Math  Operator=square  SaturateOnIntegerOverflow=on
  Math Function1 : Math  Operator=square  SaturateOnIntegerOverflow=on
  Math Function2 : Math  Operator=square  SaturateOnIntegerOverflow=on
  Square Root : Sqrt  SaturateOnIntegerOverflow=on
  Sum : Sum  Inputs=+++
  Thrust & Torque Based on Propeller Rotational and Translational Velocity : MATLAB Function  TreatAsAtomicUnit=on
  Thrust : Outport
  Resistive Torque : Outport  Port=2
  wires:
  Gain/1 -> Resistive Torque/1
  Thrust & Torque Based on Propeller Rotational and Translational Velocity/2(Torque) -> Gain/1
  Angular Speed/1 -> Thrust & Torque Based on Propeller Rotational and Translational Velocity/2(RPM)  "Speed"
  Thrust & Torque Based on Propeller Rotational and Translational Velocity/1(Thrust) -> Thrust/1
  [DX] -> Math Function/1
  Math Function/1 -> Sum/1
  Math Function2/1 -> Sum/3
  Sum/1 -> Square Root/1
  Square Root/1 -> Thrust & Torque Based on Propeller Rotational and Translational Velocity/1(Velocity)
  Math Function1/1 -> Sum/2
  [DZ] -> Math Function2/1
  [DY] -> Math Function1/1

== system Drone_Simulation/PLANT MODEL/ELECTRIC SYSTEM/Motor 5/Signals ==
  Mux : Mux  Inputs=2
      settings: DisplayOption=signals
  Spd : Outport  VectorParamsAs1DForOutWhenUnconnected=off
  ia : Outport  Port=2  VectorParamsAs1DForOutWhenUnconnected=off
  Trq : Outport  Port=3  VectorParamsAs1DForOutWhenUnconnected=off
  V : Outport  Port=4  VectorParamsAs1DForOutWhenUnconnected=off
  wires:
  [Trq5] -> Trq/1  "Motor torque [N*m]"
  [AngularSpeed5] -> Mux/2  "actual speed"
  Mux/1 -> Spd/1  "Requested and measured velocity [rpm]"
  [ReqSpeedMotor5] -> Mux/1  "req speed"
  [I_ESC_OUT5] -> ia/1  "Armature current [A]"
  [V_ESC_OUT5] -> V/1  "Motor Voltage (V)"

== system Drone_Simulation/PLANT MODEL/ELECTRIC SYSTEM/Motor 6/RPM to Resistive Torque and Thrust ==
  Angular Speed : Inport
  Gain : Gain  Gain=-1
  Math Function : Math  Operator=square  SaturateOnIntegerOverflow=on
  Math Function1 : Math  Operator=square  SaturateOnIntegerOverflow=on
  Math Function2 : Math  Operator=square  SaturateOnIntegerOverflow=on
  Square Root : Sqrt  SaturateOnIntegerOverflow=on
  Sum : Sum  Inputs=+++
  Thrust & Torque Based on Propeller Rotational and Translational Velocity : MATLAB Function  TreatAsAtomicUnit=on
  Thrust : Outport
  Resistive Torque : Outport  Port=2
  wires:
  Gain/1 -> Resistive Torque/1
  Thrust & Torque Based on Propeller Rotational and Translational Velocity/2(Torque) -> Gain/1
  Angular Speed/1 -> Thrust & Torque Based on Propeller Rotational and Translational Velocity/2(RPM)  "Speed"
  Thrust & Torque Based on Propeller Rotational and Translational Velocity/1(Thrust) -> Thrust/1
  [DX] -> Math Function/1
  Math Function/1 -> Sum/1
  Math Function2/1 -> Sum/3
  Sum/1 -> Square Root/1
  Square Root/1 -> Thrust & Torque Based on Propeller Rotational and Translational Velocity/1(Velocity)
  Math Function1/1 -> Sum/2
  [DZ] -> Math Function2/1
  [DY] -> Math Function1/1

== system Drone_Simulation/PLANT MODEL/ELECTRIC SYSTEM/Motor 6/Signals ==
  Mux : Mux  Inputs=2
      settings: DisplayOption=signals
  Spd : Outport  VectorParamsAs1DForOutWhenUnconnected=off
  ia : Outport  Port=2  VectorParamsAs1DForOutWhenUnconnected=off
  Trq : Outport  Port=3  VectorParamsAs1DForOutWhenUnconnected=off
  V : Outport  Port=4  VectorParamsAs1DForOutWhenUnconnected=off
  wires:
  [Trq6] -> Trq/1  "Motor torque [N*m]"
  [AngularSpeed6] -> Mux/2  "actual speed"
  Mux/1 -> Spd/1  "Requested and measured velocity [rpm]"
  [ReqSpeedMotor6] -> Mux/1  "req speed"
  [I_ESC_OUT6] -> ia/1  "Armature current [A]"
  [V_ESC_OUT6] -> V/1  "Motor Voltage (V)"

== system Drone_Simulation/PLANT MODEL/SENSORS/Quaternion to Rotation Angles, XYZ order/If Action Subsystem ==
  Action Port : ActionPort  ActionPortLabel=if(u1 > 1)
  Constant : Constant  SampleTime=-1
  OutputPos1 : Outport  InitialOutput=0  VectorParamsAs1DForOutWhenUnconnected=off
  wires:
  Constant/1 -> OutputPos1/1

== system Drone_Simulation/PLANT MODEL/SENSORS/Quaternion to Rotation Angles, XYZ order/If Action Subsystem1 ==
  Action Port : ActionPort  ActionPortLabel=elseif(u1 < -1)
  Constant : Constant  SampleTime=-1
  OutputNeg1 : Outport  InitialOutput=0  VectorParamsAs1DForOutWhenUnconnected=off
  wires:
  Constant/1 -> OutputNeg1/1

== system Drone_Simulation/PLANT MODEL/SENSORS/Quaternion to Rotation Angles, XYZ order/If Action Subsystem2 ==
  In : Inport
  Action Port : ActionPort  ActionPortLabel=else
  OutOrig : Outport  InitialOutput=0  VectorParamsAs1DForOutWhenUnconnected=off
  wires:
  In/1 -> OutOrig/1

== matlab function Drone_Simulation/PLANT MODEL/ELECTRIC SYSTEM/Motor 4/RPM to Resistive Torque and Thrust/Thrust & Torque Based on Propeller Rotational and Translational Velocity ==
  data: Thrust output; Velocity input; RPM input; Torque output
function [Thrust,Torque]= fcn(Velocity, RPM)

%Thrust

s1 = 0.007241;
s2 = -7.12e-05;
s3 = -0.00219;
s4 = -1.683e-05;
s5 = 1.619e-07;
Thrust = s1*Velocity + s2*RPM + s3*Velocity.^2 + s4*Velocity.*RPM + s5*RPM.^2;

%Torque

k1 = 0.000295;
k2 = -1.33e-07;
k3 = -7.089e-05;
k4 = 7.352e-08;
k5 = 2.21e-09;
Torque = k1*Velocity + k2*RPM + k3*Velocity.^2 + k4*Velocity.*RPM + k5*RPM.^2;

== matlab function Drone_Simulation/PLANT MODEL/ELECTRIC SYSTEM/Motor 5/RPM to Resistive Torque and Thrust/Thrust & Torque Based on Propeller Rotational and Translational Velocity ==
  data: Thrust output; Velocity input; RPM input; Torque output
function [Thrust,Torque]= fcn(Velocity, RPM)

%Thrust

s1 = 0.007241;
s2 = -7.12e-05;
s3 = -0.00219;
s4 = -1.683e-05;
s5 = 1.619e-07;
Thrust = s1*Velocity + s2*RPM + s3*Velocity.^2 + s4*Velocity.*RPM + s5*RPM.^2;

%Torque

k1 = 0.000295;
k2 = -1.33e-07;
k3 = -7.089e-05;
k4 = 7.352e-08;
k5 = 2.21e-09;
Torque = k1*Velocity + k2*RPM + k3*Velocity.^2 + k4*Velocity.*RPM + k5*RPM.^2;

== matlab function Drone_Simulation/PLANT MODEL/ELECTRIC SYSTEM/Motor 2/RPM to Resistive Torque and Thrust/Thrust & Torque Based on Propeller Rotational and Translational Velocity ==
  data: Thrust output; Velocity input; RPM input; Torque output
function [Thrust,Torque]= fcn(Velocity, RPM)

%Thrust

s1 = 0.007241;
s2 = -7.12e-05;
s3 = -0.00219;
s4 = -1.683e-05;
s5 = 1.619e-07;
Thrust = s1*Velocity + s2*RPM + s3*Velocity.^2 + s4*Velocity.*RPM + s5*RPM.^2;

%Torque

k1 = 0.000295;
k2 = -1.33e-07;
k3 = -7.089e-05;
k4 = 7.352e-08;
k5 = 2.21e-09;
Torque = k1*Velocity + k2*RPM + k3*Velocity.^2 + k4*Velocity.*RPM + k5*RPM.^2;

== matlab function Drone_Simulation/PLANT MODEL/ELECTRIC SYSTEM/Motor 6/RPM to Resistive Torque and Thrust/Thrust & Torque Based on Propeller Rotational and Translational Velocity ==
  data: Thrust output; Velocity input; RPM input; Torque output
function [Thrust,Torque]= fcn(Velocity, RPM)

%Thrust

s1 = 0.007241;
s2 = -7.12e-05;
s3 = -0.00219;
s4 = -1.683e-05;
s5 = 1.619e-07;
Thrust = s1*Velocity + s2*RPM + s3*Velocity.^2 + s4*Velocity.*RPM + s5*RPM.^2;

%Torque

k1 = 0.000295;
k2 = -1.33e-07;
k3 = -7.089e-05;
k4 = 7.352e-08;
k5 = 2.21e-09;
Torque = k1*Velocity + k2*RPM + k3*Velocity.^2 + k4*Velocity.*RPM + k5*RPM.^2;

== matlab function Drone_Simulation/PLANT MODEL/ELECTRIC SYSTEM/Motor 3/RPM to Resistive Torque and Thrust/Thrust & Torque Based on Propeller Rotational and Translational Velocity ==
  data: Thrust output; Velocity input; RPM input; Torque output
function [Thrust,Torque]= fcn(Velocity, RPM)

%Thrust

s1 = 0.007241;
s2 = -7.12e-05;
s3 = -0.00219;
s4 = -1.683e-05;
s5 = 1.619e-07;
Thrust = s1*Velocity + s2*RPM + s3*Velocity.^2 + s4*Velocity.*RPM + s5*RPM.^2;

%Torque

k1 = 0.000295;
k2 = -1.33e-07;
k3 = -7.089e-05;
k4 = 7.352e-08;
k5 = 2.21e-09;
Torque = k1*Velocity + k2*RPM + k3*Velocity.^2 + k4*Velocity.*RPM + k5*RPM.^2;

== matlab function Drone_Simulation/Trajectory/Trajectory Control ==
  settings: updateMethod=DISCRETE
  data: xPosition output; missionPlanX input; missionPlanY input; missionPlanZ input; missionPlanYaw input; timeConstant input; yPosition output; zPosition output; simulationTime input; yaw output
function [xPosition, yPosition, zPosition, yaw] = fcn(missionPlanX, missionPlanY, missionPlanZ, missionPlanYaw, timeConstant, simulationTime)
    persistent prevX prevY prevZ prevYaw index startTime
    if isempty(prevX)
        % Initialize the previous position, yaw, index, and timer variables
        prevX = missionPlanX(1);
        prevY = missionPlanY(1);
        prevZ = missionPlanZ(1);
        prevYaw = missionPlanYaw(1);
        index = 1;
        startTime = simulationTime;  % Record the start time
    end
    
    % Get the number of points in the mission plan
    numPoints = numel(missionPlanX);
    
    % Wrap the index within the valid range of the mission plan matrices
    if index > numPoints
        % Output the last position and yaw as signals
        xPosition = prevX;
        yPosition = prevY;
        zPosition = prevZ;
        yaw = prevYaw;
        return; % Exit the function
    end
    
    % Get the current position and yaw from the mission plan matrices
    currX = missionPlanX(index);
    currY = missionPlanY(index);
    currZ = missionPlanZ(index);
    currYaw = missionPlanYaw(index);
    
    % Calculate the Euclidean distance
    distance = sqrt((currX - prevX)^2 + (currY - prevY)^2 + (currZ - prevZ)^2+(currYaw - prevYaw)^2);
    
    % Calculate the delay time
    delay = distance * timeConstant;
    
    % Check if the elapsed time is less than the scaled delay
    elapsedTime = simulationTime - startTime;
    
    if elapsedTime < delay
        % Output the previous position and yaw as long as the delay is not reached
        xPosition = prevX;
        yPosition = prevY;
        zPosition = prevZ;
        yaw = prevYaw;
    else
        % Update the previous position and yaw
        prevX = currX;
        prevY = currY;
        prevZ = currZ;
        prevYaw = currYaw;
        
        % Update the index for the next point
        index = index + 1;
        
        % Reset the start time for the next delay
        startTime = simulationTime;
        
        % Output the current position and yaw
        xPosition = currX;
        yPosition = currY;
        zPosition = currZ;
        yaw = currYaw;
    end
end

== matlab function Drone_Simulation/PLANT MODEL/ELECTRIC SYSTEM/Motor 1/RPM to Resistive Torque and Thrust1/Thrust & Torque Based on Propeller Rotational and Translational Velocity ==
  data: Thrust output; Velocity input; RPM input; Torque output
function [Thrust,Torque]= fcn(Velocity, RPM)

%Thrust

s1 = 0.007241;
s2 = -7.12e-05;
s3 = -0.00219;
s4 = -1.683e-05;
s5 = 1.619e-07;
Thrust = s1*Velocity + s2*RPM + s3*Velocity.^2 + s4*Velocity.*RPM + s5*RPM.^2;

%Torque

k1 = 0.000295;
k2 = -1.33e-07;
k3 = -7.089e-05;
k4 = 7.352e-08;
k5 = 2.21e-09;
Torque = k1*Velocity + k2*RPM + k3*Velocity.^2 + k4*Velocity.*RPM + k5*RPM.^2;
